simulink model "taller1_simulink_v2"  (R2026a)
settings: Solver=ode45  StopTime=t_final
InitFcn:
  | run('/home/sergio/Escritorio/tdc/taller1_final/init_simulink_v2.m')
values from neighbouring files (symbols this model uses):
  dist_amp = deg2rad(1.0)    [init_simulink.m]    (also in init_simulink_v2.m)
  dist_enabled = 1    [init_simulink_v2.m]
  dist_freq = 2*pi*6    (= 37.6991118431)    [init_simulink.m]    (also in init_simulink_v2.m)
  n_Kphi = size(Kphi_A, 1)    [init_simulink_v2.m]
  n_Ktheta = size(Ktheta_A, 1)    [init_simulink_v2.m]
  n_p = size(Gp_A, 1)    [init_simulink_v2.m]
  n_phi = size(Gphi_A, 1)    [init_simulink_v2.m]
  n_q = size(Gq_A, 1)    [init_simulink_v2.m]
  n_theta = size(Gtheta_A, 1)    [init_simulink_v2.m]
  noise_enabled = 1    [init_simulink_v2.m]
  noise_power_lat = 1e-3    (= 0.001)    [init_simulink.m]    (also in init_simulink_v2.m; taller1_completo.m)
  noise_power_long = 1e-4    (= 0.0001)    [init_simulink.m]    (also in init_simulink_v2.m; taller1_completo.m)
  noise_sample_time = 0.005    [init_simulink.m]    (also in init_simulink_v2.m)
  sas_D_p = kd_phi    (= 0.05)    [init_simulink.m]    (also in init_simulink_v2.m)
  sas_D_q = kd_theta    (= -0.2)    [init_simulink.m]    (also in init_simulink_v2.m)
  t_step = 1.0    (= 1)    [init_simulink.m]    (also in init_simulink_v2.m; taller1_completo.m)
  umax = deg2rad(control_limit_deg)    [init_simulink.m]    (also in init_simulink_v2.m)
undefined symbols (not defined in the file or in its folder): cas_pi_phi_den, cas_pi_phi_num, cas_pi_theta_den, cas_pi_theta_num, Gp_A, Gp_B, Gp_C, Gp_D, Gphi_A, Gphi_B, Gphi_C, Gphi_D, Gq_A, Gq_B, Gq_C, Gq_D, Gtheta_A, Gtheta_B, Gtheta_C, Gtheta_D, Kphi_A, Kphi_B, Kphi_C, Kphi_D, Ktheta_A, Ktheta_B, Ktheta_C, Ktheta_D, Kyaw_A, Kyaw_B, Kyaw_C, Kyaw_D
settings Model: Creator=sergio  LastModifiedBy=sergio

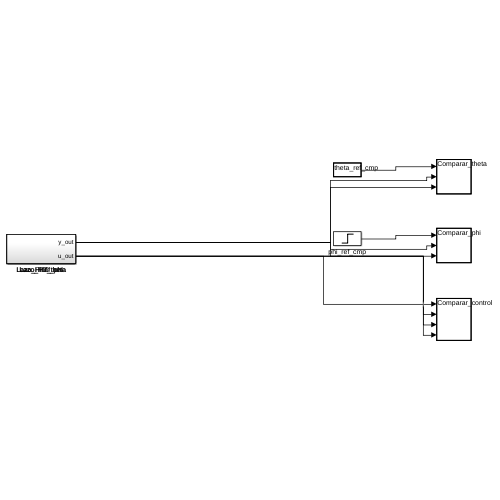
[thumbnail: Simulink's stored preview of the top-level diagram]
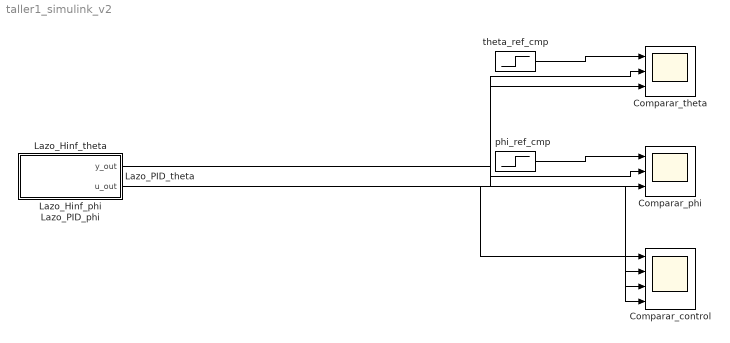
== system taller1_simulink_v2 ==
  Comparar_control : Scope  NumInputPorts=4
  Comparar_phi : Scope  NumInputPorts=3
  Comparar_theta : Scope  NumInputPorts=3
  Lazo_Hinf_phi : Subsystem
  Lazo_Hinf_theta : Subsystem
  Lazo_PID_phi : Subsystem
  Lazo_PID_theta : Subsystem
  phi_ref_cmp : Step  Time=t_step  FinalValue=phi_ref_amp  SampleTime=0
  theta_ref_cmp : Step  Time=t_step  FinalValue=theta_ref_amp  SampleTime=0
  wires:
  theta_ref_cmp/1 -> Comparar_theta/1
  Lazo_PID_theta/1(y_out) -> Comparar_theta/2
  Lazo_Hinf_theta/1(y_out) -> Comparar_theta/3
  phi_ref_cmp/1 -> Comparar_phi/1
  Lazo_PID_phi/1(y_out) -> Comparar_phi/2
  Lazo_Hinf_phi/1(y_out) -> Comparar_phi/3
  Lazo_PID_theta/2(u_out) -> Comparar_control/1
  Lazo_Hinf_theta/2(u_out) -> Comparar_control/2
  Lazo_PID_phi/2(u_out) -> Comparar_control/3
  Lazo_Hinf_phi/2(u_out) -> Comparar_control/4

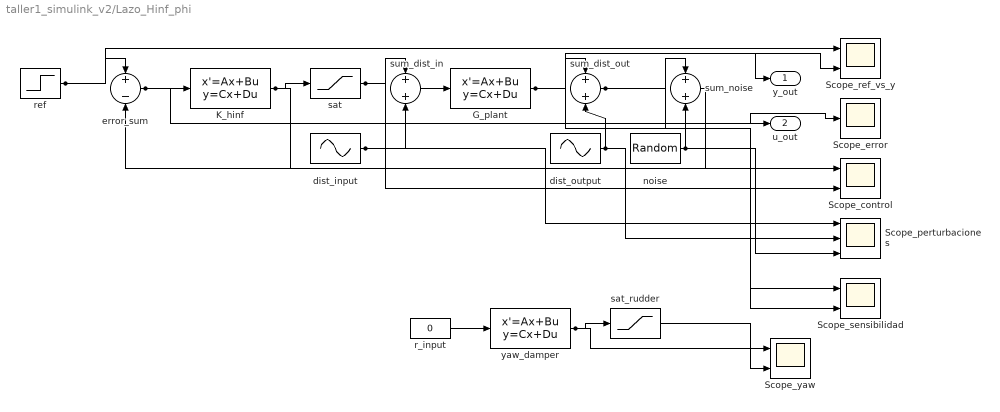
== system taller1_simulink_v2/Lazo_Hinf_phi ==
  G_plant : StateSpace  A=Gphi_A  B=Gphi_B  C=Gphi_C  D=Gphi_D  InitialCondition=zeros(n_phi,1)
  K_hinf : StateSpace  A=Kphi_A  B=Kphi_B  C=Kphi_C  D=Kphi_D  InitialCondition=zeros(n_Kphi,1)
  Scope_control : Scope  NumInputPorts=2
  Scope_error : Scope
  Scope_perturbaciones : Scope  NumInputPorts=3
  Scope_ref_vs_y : Scope  NumInputPorts=2
  Scope_sensibilidad : Scope  NumInputPorts=2
  Scope_yaw : Scope  NumInputPorts=2
  dist_input : Sin  Amplitude=dist_amp*dist_enabled  Frequency=dist_freq  SampleTime=0
  dist_output : Sin  Amplitude=dist_amp*dist_enabled*0.5  Frequency=dist_freq*1.5  SampleTime=0
  error_sum : Sum  Inputs=+-
  noise : RandomNumber  Variance=noise_power_lat*noise_enabled  Seed=13  SampleTime=noise_sample_time
  r_input : Constant  Value=0
  ref : Step  Time=t_step  FinalValue=phi_ref_amp  SampleTime=0
  sat : Saturate  UpperLimit=umax  LowerLimit=-umax
  sat_rudder : Saturate  UpperLimit=umax  LowerLimit=-umax
  sum_dist_in : Sum
  sum_dist_out : Sum
  sum_noise : Sum
  yaw_damper : StateSpace  A=Kyaw_A  B=Kyaw_B  C=Kyaw_C  D=Kyaw_D  InitialCondition=0
  y_out : Outport
  u_out : Outport  Port=2
  wires:
  ref/1 -> error_sum/1, Scope_ref_vs_y/1
  error_sum/1 -> K_hinf/1, Scope_error/1
  K_hinf/1 -> sat/1, Scope_control/1
  sat/1 -> sum_dist_in/1, u_out/1, Scope_control/2
  dist_input/1 -> sum_dist_in/2, Scope_perturbaciones/1
  sum_dist_in/1 -> G_plant/1
  G_plant/1 -> sum_dist_out/1, y_out/1, Scope_ref_vs_y/2, Scope_sensibilidad/2
  dist_output/1 -> sum_dist_out/2, Scope_perturbaciones/2
  sum_dist_out/1 -> sum_noise/1, Scope_sensibilidad/1
  noise/1 -> sum_noise/2, Scope_perturbaciones/3
  sum_noise/1 -> error_sum/2
  r_input/1 -> yaw_damper/1
  yaw_damper/1 -> sat_rudder/1, Scope_yaw/1
  sat_rudder/1 -> Scope_yaw/2

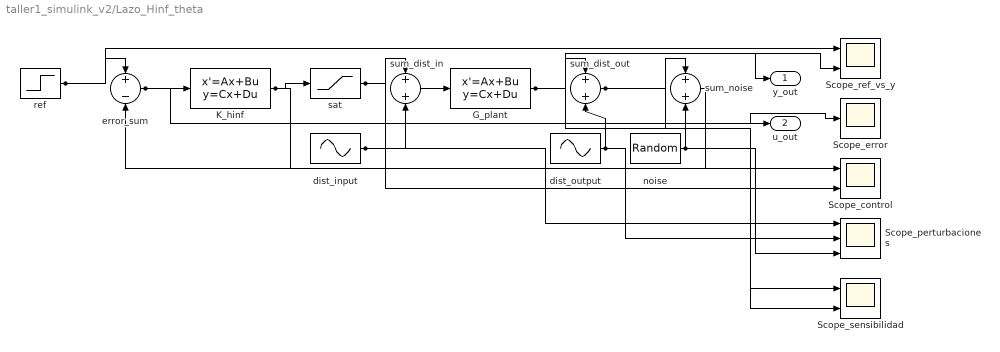
== system taller1_simulink_v2/Lazo_Hinf_theta ==
  G_plant : StateSpace  A=Gtheta_A  B=Gtheta_B  C=Gtheta_C  D=Gtheta_D  InitialCondition=zeros(n_theta,1)
  K_hinf : StateSpace  A=Ktheta_A  B=Ktheta_B  C=Ktheta_C  D=Ktheta_D  InitialCondition=zeros(n_Ktheta,1)
  Scope_control : Scope  NumInputPorts=2
  Scope_error : Scope
  Scope_perturbaciones : Scope  NumInputPorts=3
  Scope_ref_vs_y : Scope  NumInputPorts=2
  Scope_sensibilidad : Scope  NumInputPorts=2
  dist_input : Sin  Amplitude=dist_amp*dist_enabled  Frequency=dist_freq  SampleTime=0
  dist_output : Sin  Amplitude=dist_amp*dist_enabled*0.5  Frequency=dist_freq*1.5  SampleTime=0
  error_sum : Sum  Inputs=+-
  noise : RandomNumber  Variance=noise_power_long*noise_enabled  Seed=13  SampleTime=noise_sample_time
  ref : Step  Time=t_step  FinalValue=theta_ref_amp  SampleTime=0
  sat : Saturate  UpperLimit=umax  LowerLimit=-umax
  sum_dist_in : Sum
  sum_dist_out : Sum
  sum_noise : Sum
  y_out : Outport
  u_out : Outport  Port=2
  wires:
  ref/1 -> error_sum/1, Scope_ref_vs_y/1
  error_sum/1 -> K_hinf/1, Scope_error/1
  K_hinf/1 -> sat/1, Scope_control/1
  sat/1 -> sum_dist_in/1, u_out/1, Scope_control/2
  dist_input/1 -> sum_dist_in/2, Scope_perturbaciones/1
  sum_dist_in/1 -> G_plant/1
  G_plant/1 -> sum_dist_out/1, y_out/1, Scope_ref_vs_y/2, Scope_sensibilidad/2
  dist_output/1 -> sum_dist_out/2, Scope_perturbaciones/2
  sum_dist_out/1 -> sum_noise/1, Scope_sensibilidad/1
  noise/1 -> sum_noise/2, Scope_perturbaciones/3
  sum_noise/1 -> error_sum/2

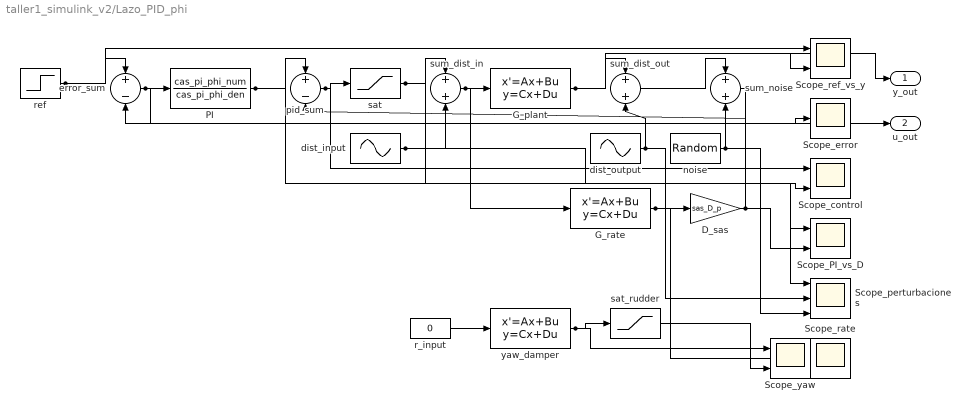
== system taller1_simulink_v2/Lazo_PID_phi ==
  D_sas : Gain  Gain=sas_D_p
  G_plant : StateSpace  A=Gphi_A  B=Gphi_B  C=Gphi_C  D=Gphi_D  InitialCondition=zeros(n_phi,1)
  G_rate : StateSpace  A=Gp_A  B=Gp_B  C=Gp_C  D=Gp_D  InitialCondition=zeros(n_p,1)
  PI : TransferFcn  Numerator=cas_pi_phi_num  Denominator=cas_pi_phi_den
  Scope_PI_vs_D : Scope  NumInputPorts=2
  Scope_control : Scope  NumInputPorts=2
  Scope_error : Scope
  Scope_perturbaciones : Scope  NumInputPorts=3
  Scope_rate : Scope
  Scope_ref_vs_y : Scope  NumInputPorts=2
  Scope_yaw : Scope  NumInputPorts=2
  dist_input : Sin  Amplitude=dist_amp*dist_enabled  Frequency=dist_freq  SampleTime=0
  dist_output : Sin  Amplitude=dist_amp*dist_enabled*0.5  Frequency=dist_freq*1.5  SampleTime=0
  error_sum : Sum  Inputs=+-
  noise : RandomNumber  Variance=noise_power_lat*noise_enabled  Seed=11  SampleTime=noise_sample_time
  pid_sum : Sum  Inputs=+-
  r_input : Constant  Value=0
  ref : Step  Time=t_step  FinalValue=phi_ref_amp  SampleTime=0
  sat : Saturate  UpperLimit=umax  LowerLimit=-umax
  sat_rudder : Saturate  UpperLimit=umax  LowerLimit=-umax
  sum_dist_in : Sum
  sum_dist_out : Sum
  sum_noise : Sum
  yaw_damper : StateSpace  A=Kyaw_A  B=Kyaw_B  C=Kyaw_C  D=Kyaw_D  InitialCondition=0
  y_out : Outport
  u_out : Outport  Port=2
  wires:
  ref/1 -> error_sum/1, Scope_ref_vs_y/1
  error_sum/1 -> PI/1, Scope_error/1
  PI/1 -> pid_sum/1, Scope_PI_vs_D/1
  D_sas/1 -> pid_sum/2, Scope_PI_vs_D/2
  pid_sum/1 -> sat/1, Scope_control/1
  sat/1 -> sum_dist_in/1, u_out/1, Scope_control/2
  dist_input/1 -> sum_dist_in/2, Scope_perturbaciones/1
  sum_dist_in/1 -> G_plant/1, G_rate/1
  G_rate/1 -> D_sas/1, Scope_rate/1
  G_plant/1 -> sum_dist_out/1, y_out/1, Scope_ref_vs_y/2
  dist_output/1 -> sum_dist_out/2, Scope_perturbaciones/2
  sum_dist_out/1 -> sum_noise/1
  noise/1 -> sum_noise/2, Scope_perturbaciones/3
  sum_noise/1 -> error_sum/2
  r_input/1 -> yaw_damper/1
  yaw_damper/1 -> sat_rudder/1, Scope_yaw/1
  sat_rudder/1 -> Scope_yaw/2

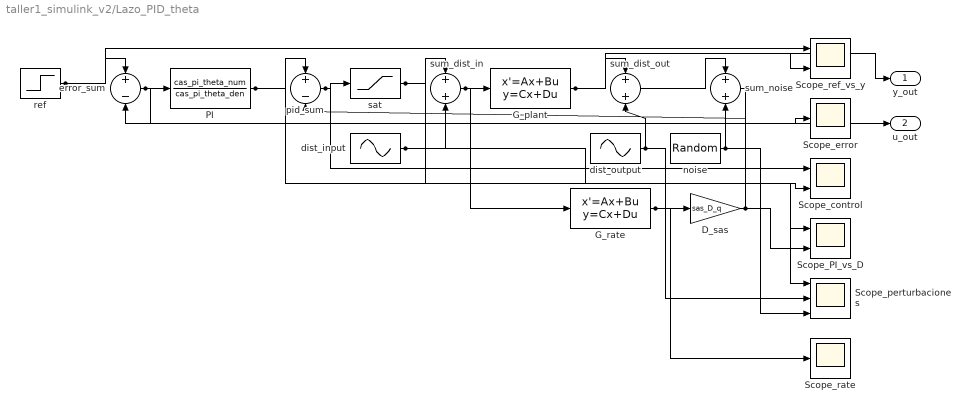
== system taller1_simulink_v2/Lazo_PID_theta ==
  D_sas : Gain  Gain=sas_D_q
  G_plant : StateSpace  A=Gtheta_A  B=Gtheta_B  C=Gtheta_C  D=Gtheta_D  InitialCondition=zeros(n_theta,1)
  G_rate : StateSpace  A=Gq_A  B=Gq_B  C=Gq_C  D=Gq_D  InitialCondition=zeros(n_q,1)
  PI : TransferFcn  Numerator=cas_pi_theta_num  Denominator=cas_pi_theta_den
  Scope_PI_vs_D : Scope  NumInputPorts=2
  Scope_control : Scope  NumInputPorts=2
  Scope_error : Scope
  Scope_perturbaciones : Scope  NumInputPorts=3
  Scope_rate : Scope
  Scope_ref_vs_y : Scope  NumInputPorts=2
  dist_input : Sin  Amplitude=dist_amp*dist_enabled  Frequency=dist_freq  SampleTime=0
  dist_output : Sin  Amplitude=dist_amp*dist_enabled*0.5  Frequency=dist_freq*1.5  SampleTime=0
  error_sum : Sum  Inputs=+-
  noise : RandomNumber  Variance=noise_power_long*noise_enabled  Seed=11  SampleTime=noise_sample_time
  pid_sum : Sum  Inputs=+-
  ref : Step  Time=t_step  FinalValue=theta_ref_amp  SampleTime=0
  sat : Saturate  UpperLimit=umax  LowerLimit=-umax
  sum_dist_in : Sum
  sum_dist_out : Sum
  sum_noise : Sum
  y_out : Outport
  u_out : Outport  Port=2
  wires:
  ref/1 -> error_sum/1, Scope_ref_vs_y/1
  error_sum/1 -> PI/1, Scope_error/1
  PI/1 -> pid_sum/1, Scope_PI_vs_D/1
  D_sas/1 -> pid_sum/2, Scope_PI_vs_D/2
  pid_sum/1 -> sat/1, Scope_control/1
  sat/1 -> sum_dist_in/1, u_out/1, Scope_control/2
  dist_input/1 -> sum_dist_in/2, Scope_perturbaciones/1
  sum_dist_in/1 -> G_plant/1, G_rate/1
  G_rate/1 -> D_sas/1, Scope_rate/1
  G_plant/1 -> sum_dist_out/1, y_out/1, Scope_ref_vs_y/2
  dist_output/1 -> sum_dist_out/2, Scope_perturbaciones/2
  sum_dist_out/1 -> sum_noise/1
  noise/1 -> sum_noise/2, Scope_perturbaciones/3
  sum_noise/1 -> error_sum/2
